simulink model "Identification_Phase_Model"  (R2025b)
settings: Solver=ode4  StartTime=0.0  StopTime=10  FixedStep=0.001  RelTol=1e-3
undefined symbols (not defined in the file): b, j, km, l, mu, r
settings Model: Creator=moata  LastModifiedBy=moata
settings DataIOCC: ReturnWorkspaceOutputs=off

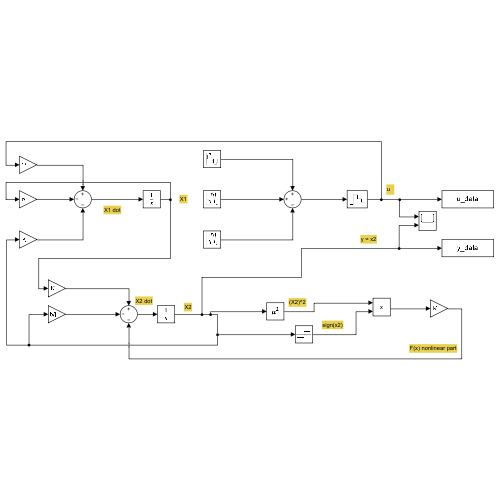
[thumbnail: Simulink's stored preview of the top-level diagram]
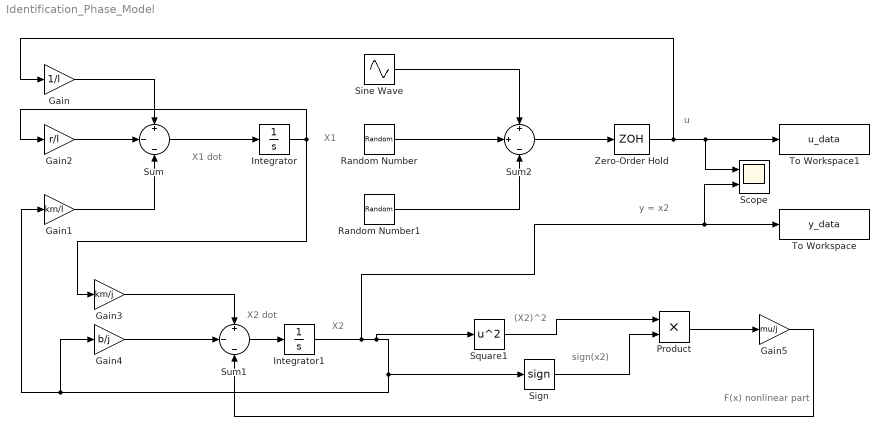
== system Identification_Phase_Model ==
  note: X1 dot
  note: X1
  note: X2 dot
  note: X2
  note: u
  note: y = x2
  note: F(x) nonlinear part
  note: (X2)^2
  note: sign(x2)
  Gain : Gain  Gain=1/l
  Gain1 : Gain  Gain=km/l
  Gain2 : Gain  Gain=r/l
  Gain3 : Gain  Gain=km/j
  Gain4 : Gain  Gain=b/j
  Gain5 : Gain  Gain=mu/j
  Integrator : Integrator
  Integrator1 : Integrator
  Product : Product
  Random Number : RandomNumber  Mean=0.5  Variance=1/12  SampleTime=0.04
  Random Number1 : RandomNumber  Mean=0.5  Variance=1/12  SampleTime=0.04
  Scope : Scope  NumInputPorts=2
      settings: ActiveDisplayYMinimum=-49.942814735524273  ActiveDisplayYMaximum=49.939728355028542
  Sign : Signum
  Sine Wave : Sin  Amplitude=40  Frequency=3.14  SampleTime=0.04
  Square1 : Math  Operator=square
  Sum : Sum  Inputs=+|-|-
  Sum1 : Sum  Inputs=+|-|-
  Sum2 : Sum  Inputs=+|+|-
  To Workspace : ToWorkspace  VariableName=y_data  SampleTime=0.04
  To Workspace1 : ToWorkspace  VariableName=u_data  SampleTime=0.04
  Zero-Order Hold : ZeroOrderHold  SampleTime=0.04
  wires:
  Sum/1 -> Integrator/1
  Gain/1 -> Sum/1
  Gain2/1 -> Sum/2
  Gain1/1 -> Sum/3
  Gain3/1 -> Sum1/1
  Integrator/1 -> Gain2/1, Gain3/1
  Gain4/1 -> Sum1/2
  Integrator1/1 -> Scope/2, To Workspace/1, Square1/1, Sign/1, Gain4/1, Gain1/1
  Sign/1 -> Product/2
  Square1/1 -> Product/1
  Product/1 -> Gain5/1
  Gain5/1 -> Sum1/3
  Sine Wave/1 -> Sum2/1
  Random Number/1 -> Sum2/2
  Random Number1/1 -> Sum2/3
  Sum2/1 -> Zero-Order Hold/1
  Zero-Order Hold/1 -> To Workspace1/1, Scope/1, Gain/1
  Sum1/1 -> Integrator1/1
